simulink model "fuzzyControllerTestBench"  (R2013b)
settings: Solver=FixedStepDiscrete  StartTime=0.0  StopTime=10  RelTol=1e-3
libraries: fuzblock x1
settings Model: NumberOfSteps=1000  Creator=Raj  LastModifiedBy=Raj
settings OptimizationCC: UseIntDivNetSlope=on  UseFloatMulNetSlope=on  EfficientMapNaN2IntZero=off  OptimizeModelRefInitCode=on  LifeSpan=1  MaxStackSize=64
settings DebuggingCC: ConsistencyChecking=warning  TimeAdjustmentMsg=warning  StateNameClashWarn=warning
settings HardwareCC: ProdLargestAtomicInteger=Long  ProdLargestAtomicFloat=Double  ProdEndianess=LittleEndian  ProdHWDeviceType=ARM Compatible->ARM Cortex
settings RTWCC: SystemTargetFile=ert.tlc  GenCodeOnly=on  TemplateMakefile=ert_default_tmf  Description=Embedded Coder  ProcessScript=ert_make_rtw_hook  Toolchain=GNU Tools for ARM Embedded Processors
settings CodeAppCC: IgnoreCustomStorageClasses=off
settings ERTTargetCC: CodeReplacementLibrary=C89/C90 (ANSI)  IncludeMdlTerminateFcn=off  SuppressErrorStatus=on  SupportNonFinite=off  ERTCustomFileTemplate=example_file_process.tlc  ERTFilePackagingFormat=CompactWithDataFile  ConvertIfToSwitch=on

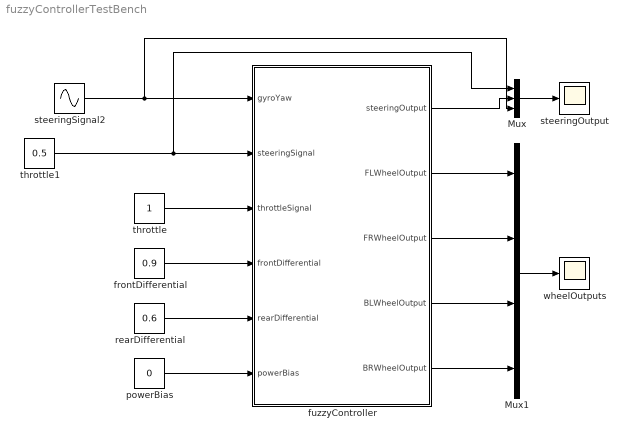
== system fuzzyControllerTestBench ==
  Mux : Mux  Inputs=3
  Mux1 : Mux
  frontDifferential : Constant  Value=0.9
  fuzzyController : Subsystem
  powerBias : Constant  Value=0
  rearDifferential : Constant  Value=0.6
  steeringOutput : Scope
  steeringSignal2 : Sin  Amplitude=0.5  Frequency=8  SampleTime=0
  throttle : Constant
  throttle1 : Constant  Value=0.5
  wheelOutputs : Scope
  wires:
  frontDifferential/1 -> fuzzyController/4(frontDifferential)
  rearDifferential/1 -> fuzzyController/5(rearDifferential)
  powerBias/1 -> fuzzyController/6(powerBias)
  fuzzyController/2(FLWheelOutput) -> Mux1/1
  fuzzyController/5(BRWheelOutput) -> Mux1/4
  fuzzyController/1(steeringOutput) -> Mux/2
  Mux/1 -> steeringOutput/1
  fuzzyController/4(BLWheelOutput) -> Mux1/3
  fuzzyController/3(FRWheelOutput) -> Mux1/2
  Mux1/1 -> wheelOutputs/1
  throttle/1 -> fuzzyController/3(throttleSignal)
  throttle1/1 -> Mux/1, fuzzyController/2(steeringSignal)
  steeringSignal2/1 -> Mux/3, fuzzyController/1(gyroYaw)

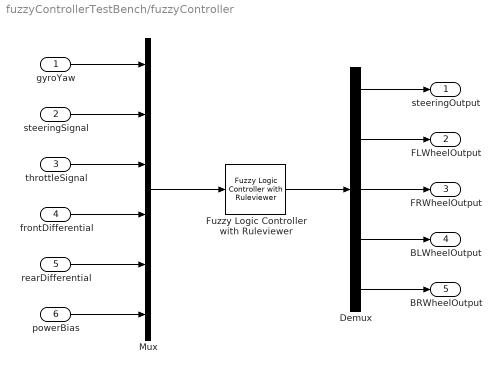
== system fuzzyControllerTestBench/fuzzyController ==
  gyroYaw : Inport  OutDataTypeStr=double
  steeringSignal : Inport  Port=2  OutDataTypeStr=double
  throttleSignal : Inport  Port=3  OutDataTypeStr=double
  frontDifferential : Inport  Port=4  OutDataTypeStr=double
  rearDifferential : Inport  Port=5  OutDataTypeStr=double
  powerBias : Inport  Port=6  OutDataTypeStr=double
  Demux : Demux  Outputs=5
  Fuzzy Logic Controller with Ruleviewer : fuzblock/Fuzzy Logic  Controller  with Ruleviewer  fismatrix=fuzzyController  Ts=0.01
  Mux : Mux  Inputs=6
  steeringOutput : Outport  OutDataTypeStr=double
  FLWheelOutput : Outport  Port=2  OutDataTypeStr=double
  FRWheelOutput : Outport  Port=3  OutDataTypeStr=double
  BLWheelOutput : Outport  Port=4  OutDataTypeStr=double
  BRWheelOutput : Outport  Port=5  OutDataTypeStr=double
  wires:
  gyroYaw/1 -> Mux/1
  steeringSignal/1 -> Mux/2
  frontDifferential/1 -> Mux/4
  Fuzzy Logic Controller with Ruleviewer/1 -> Demux/1
  powerBias/1 -> Mux/6
  Demux/4 -> BLWheelOutput/1
  Demux/3 -> FRWheelOutput/1
  Demux/1 -> steeringOutput/1
  Demux/2 -> FLWheelOutput/1
  Demux/5 -> BRWheelOutput/1
  rearDifferential/1 -> Mux/5
  throttleSignal/1 -> Mux/3
  Mux/1 -> Fuzzy Logic Controller with Ruleviewer/1
